simulink model "PSK"  (R2024a)
settings: Solver=VariableStepAuto  StartTime=0.0  StopTime=10.0  RelTol=1e-3
settings Model: Creator=prath  LastModifiedBy=prath

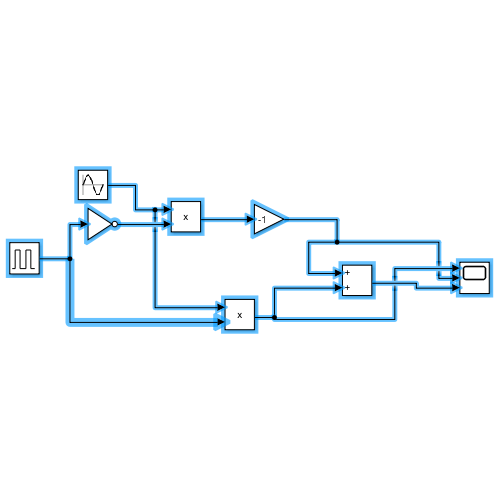
[thumbnail: Simulink's stored preview of the top-level diagram]
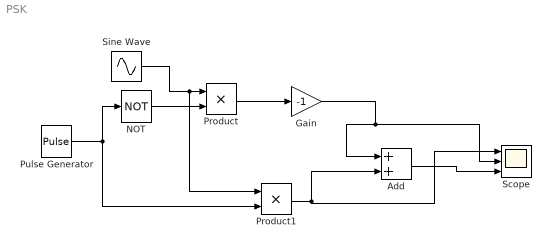
== system PSK ==
  Add : Sum
  Gain : Gain  Gain=-1
  NOT : Logic  Operator=NOT  IconShape=distinctive  AllPortsSameDT=off  OutDataTypeStr=boolean
  Product : Product
  Product1 : Product
  Pulse Generator : DiscretePulseGenerator  PulseType=Time based  PulseWidth=50
  Scope : Scope  NumInputPorts=3
  Sine Wave : Sin  Frequency=50  SampleTime=0
  wires:
  Gain/1 -> Add/1, Scope/2
  Sine Wave/1 -> Product1/1, Product/1
  Add/1 -> Scope/3
  NOT/1 -> Product/2
  Product/1 -> Gain/1
  Product1/1 -> Scope/1, Add/2
  Pulse Generator/1 -> Product1/2, NOT/1
